simulink library "angleBtw2Vecs_ul"  (R2018b)
settings: Solver=VariableStepAuto  StartTime=0.0  StopTime=10.0  RelTol=1e-3
settings Model: Creator=James Reed  LastModifiedBy=mcobb

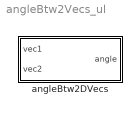
== system angleBtw2Vecs_ul ==
  angleBtw2DVecs : Subsystem

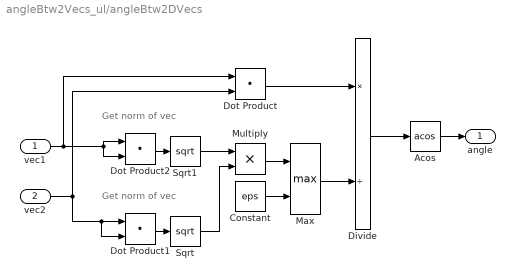
== system angleBtw2Vecs_ul/angleBtw2DVecs ==
  note: Get norm of vec
  note: Get norm of vec
  vec1 : Inport
  vec2 : Inport  Port=2
  Acos : Trigonometry  Operator=acos
  Constant : Constant  Value=eps
  Divide : Product  Inputs=*/
  Dot Product : DotProduct  InputSameDT=on  OutDataTypeStr=Inherit: Inherit via internal rule
  Dot Product1 : DotProduct  InputSameDT=on  OutDataTypeStr=Inherit: Inherit via internal rule
  Dot Product2 : DotProduct  InputSameDT=on  OutDataTypeStr=Inherit: Inherit via internal rule
  Max : MinMax  Function=max  Inputs=2
  Multiply : Product
  Sqrt : Sqrt  SaturateOnIntegerOverflow=on
  Sqrt1 : Sqrt  SaturateOnIntegerOverflow=on
  angle : Outport
  wires:
  Divide/1 -> Acos/1
  Dot Product/1 -> Divide/1
  Acos/1 -> angle/1
  Dot Product1/1 -> Sqrt/1
  Sqrt/1 -> Multiply/2
  vec1/1 -> Dot Product/1, Dot Product2/2, Dot Product2/1
  Sqrt1/1 -> Multiply/1
  Dot Product2/1 -> Sqrt1/1
  vec2/1 -> Dot Product/2, Dot Product1/2, Dot Product1/1
  Multiply/1 -> Max/1
  Constant/1 -> Max/2
  Max/1 -> Divide/2
